simulink model "closed_loop_8room_sim"  (R2022b)
settings: Solver=VariableStepAuto  StartTime=0.0  StopTime=30000  RelTol=1e-3
values from neighbouring files (symbols this model uses):
  A = A .* (1 ./ capacs)    [closed_loop_8rooms.m]    (also in closed_loop_control.m = 100*[-1/capacA * (htAO + htAB + htAC), htAB / capacA,       ; control_time_dependent_A.m = 100*[-1/capacA * (htAO + htAB + htAC), htAB / capacA,       ; open_loop_8rooms.m; open_loop_control.m = 100*[-1/capacA * (htAO + htAB + htAC), htAB / capacA,       )
  B = diag([0 1 0 1 0 1 1 1]) .* (1 ./ capacs)    [closed_loop_8rooms.m]    (also in closed_loop_control.m = [1 / capacA, 0, 0; 0, 1/capacB, 0; 0, 0, 1/capacC]; control_time_dependent_A.m = [1 / capacA, 0, 0; 0, 1/capacB, 0; 0, 0, 1/capacC]; open_loop_8rooms.m; open_loop_control.m = [1 / capacA, 0, 0; 0, 1/capacB, 0; 0, 0, 1/capacC])
  C = diag([0 1 0 1 1 0 0 1])    [closed_loop_8rooms.m]    (also in closed_loop_control.m = [1, 0, 0; 1, 0, 0; 1, 0, 0]; control_time_dependent_A.m = [1, 0, 0; 0, 1, 0; 0, 0, 1]; open_loop_8rooms.m = eye(8); open_loop_control.m = [1, 0, 0; 0, 1, 0; 0, 0, 1])
  D = zeros(8, 8)    [closed_loop_8rooms.m]    (also in closed_loop_control.m = [0, 0, 0; 0, 0, 0; 0, 0, 0]; control_time_dependent_A.m = [0, 0, 0; 0, 0, 0; 0, 0, 0]; open_loop_8rooms.m; open_loop_control.m = [0, 0, 0; 0, 0, 0; 0, 0, 0])
  u_des = -pinv(A\B)*x_des    [closed_loop_8rooms.m]    (also in closed_loop_control.m)
  x0 = [0;0;0;0;0;0;0;0]    [closed_loop_8rooms.m]    (also in closed_loop_control.m = [0;0;0]; control_time_dependent_A.m = [0,0,0]; open_loop_8rooms.m = zeros(8, 1); open_loop_control.m = [0; 0; 0])
  x_des = [20;20;20;20;20;20;20;20]    [closed_loop_8rooms.m]    (also in closed_loop_control.m = [20;20;20]; control_time_dependent_A.m = [20; 20; 20]; open_loop_8rooms.m = [20; 20; 20; 20; 20; 20; 20; 20]; open_loop_control.m = [20; 20; 20])
undefined symbols (not defined in the file or in its folder): K
settings Model: Creator=dahliasaba  LastModifiedBy=corlenerhoades
settings OptimizationCC: ReuseModelBlockBuffer=on

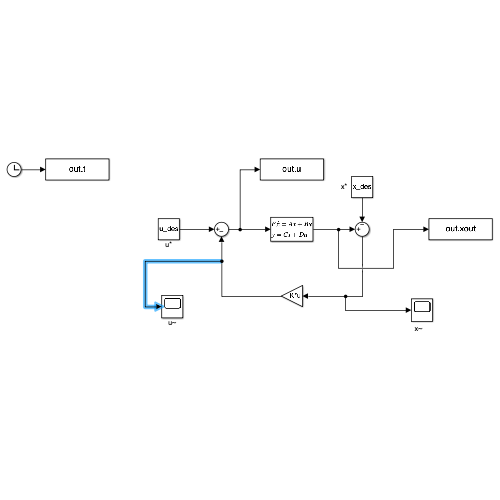
[thumbnail: Simulink's stored preview of the top-level diagram]
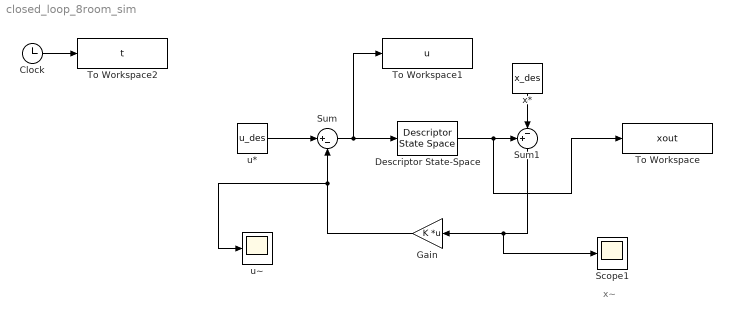
== system closed_loop_8room_sim ==
  note: x~
  Clock : Clock
  Descriptor State-Space : DescriptorStateSpace  E=eye(8)  A=A  B=B  C=C  D=D  InitialCondition=x0
  Gain : Gain  Gain=K  Multiplication=Matrix(K*u)
  Scope1 : Scope
  Sum : Sum  Inputs=|+-
  Sum1 : Sum  Inputs=+-|
  To Workspace : ToWorkspace  VariableName=xout  SampleTime=-1
  To Workspace1 : ToWorkspace  VariableName=u  SampleTime=-1
  To Workspace2 : ToWorkspace  VariableName=t  SampleTime=-1
  u* : Constant  Value=u_des
  u~ : Scope
  x* : Constant  Value=x_des
  wires:
  u*/1 -> Sum/1
  Sum/1 -> To Workspace1/1, Descriptor State-Space/1
  Gain/1 -> u~/1, Sum/2
  Descriptor State-Space/1 -> To Workspace/1, Sum1/1
  x*/1 -> Sum1/2
  Sum1/1 -> Scope1/1, Gain/1
  Clock/1 -> To Workspace2/1
